simulink model "sampleModel185"  (R2021b)
settings: Solver=VariableStepAuto  StartTime=0.0  StopTime=10.0  RelTol=1e-3
undefined symbols (not defined in the file or in its folder): DiscIntNeverNeededParam, Newton, Raphson
libraries: simulink x18, slpidlib x1
settings Model: Creator=user  LastModifiedBy=user

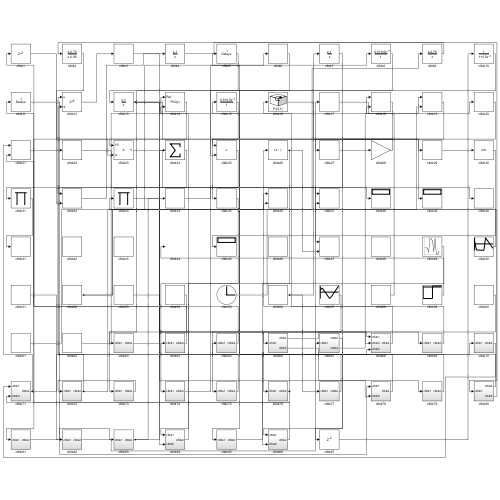
[thumbnail: Simulink's stored preview of the top-level diagram]
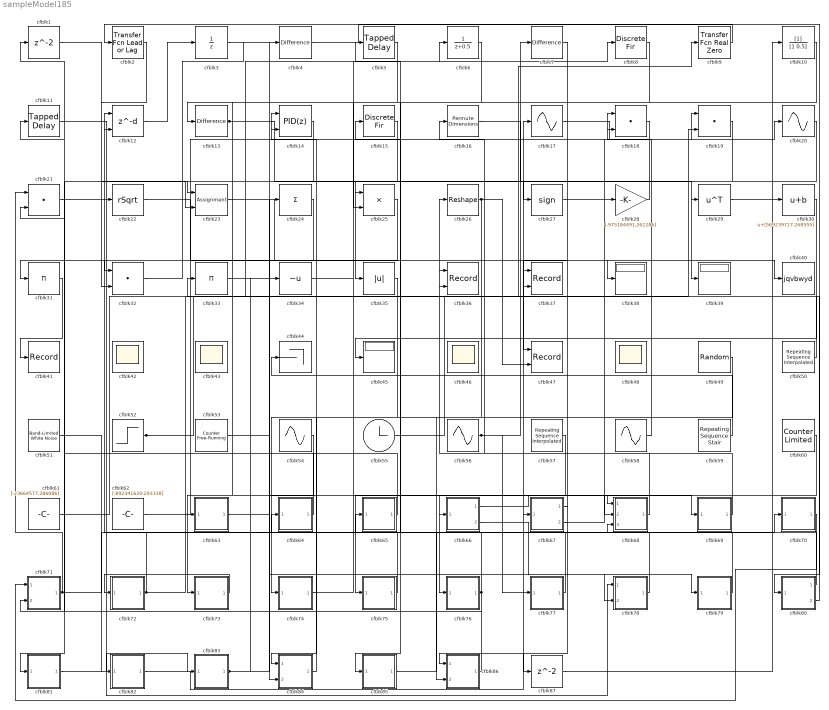
== system sampleModel185 ==
  cfblk1 : Delay  SampleTime=1
  cfblk10 : DiscreteFilter  SampleTime=1
  cfblk11 : simulink/Discrete/Tapped Delay  vinit=0.0  samptime=-1  NumDelays=1  DelayOrder=Oldest  includeCurrent=off
  cfblk12 : Delay  DelayLengthSource=Input port  SampleTime=1
      settings: InputPortMap=u0,p1
  cfblk13 : simulink/Discrete/Difference  ICPrevInput=0.0  OutMin=[]  OutMax=[]  OutDataTypeStr=Inherit: Inherit via back propagation  OutDataType=fixdt(1, 16)  OutScaling=2^-10  DoSatur=off
  cfblk14 : slpidlib/PID Controller (2DOF)  Controller=PID  Form=Parallel  TimeDomain=Discrete-time  UseExternalTs=off  SampleTime=1  IntegratorMethod=Forward Euler  FilterMethod=Forward Euler  ControllerParametersSource=internal  P=1  I=1  D=0  UseFilter=on  N=100  b=1  c=1  TunerSelectOption=Transfer Function Based (PID Tuner App)  InitialConditionSource=internal  InitialConditionForIntegrator=0  InitialConditionForFilter=0  DifferentiatorICPrevScaledInput=0  ExternalReset=none  TrackingMode=off  Kt=1  LimitOutput=off  SatLimitsSource=internal  UpperSaturationLimit=inf  LowerSaturationLimit=-inf  LinearizeAsGain=off  AntiWindupMode=none  Kb=1  POutMin=[]  POutMax=[]  IOutMin=[]  IOutMax=[]  DOutMin=[]  DOutMax=[]  NOutMin=[]  NOutMax=[]  bOutMin=[]  bOutMax=[]  cOutMin=[]  cOutMax=[]  SumOutMin=[]  SumOutMax=[]  SaturationOutMin=[]  SaturationOutMax=[]  PParamMin=[]  PParamMax=[]  IParamMin=[]  IParamMax=[]  DParamMin=[]  DParamMax=[]  NParamMin=[]  NParamMax=[]  bParamMin=[]  bParamMax=[]  cParamMin=[]  cParamMax=[]  KbParamMin=[]  KbParamMax=[]  KtParamMin=[]  KtParamMax=[]  KbOutMin=[]  KbOutMax=[]  KtOutMin=[]  KtOutMax=[]  IntegratorOutMin=[]  IntegratorOutMax=[]  FilterOutMin=[]  FilterOutMax=[]  SumI1OutMin=[]  SumI1OutMax=[]  SumI2OutMin=[]  SumI2OutMax=[]  SumI3OutMin=[]  SumI3OutMax=[]  SumI4OutMin=[]  SumI4OutMax=[]  SumDOutMin=[]  SumDOutMax=[]  Sum1OutMin=[]  Sum1OutMax=[]  Sum2OutMin=[]  Sum2OutMax=[]  Sum3OutMin=[]  Sum3OutMax=[]  DifferentiatorOutMin=[]  DifferentiatorOutMax=[]  FilterDiffOutCoefMin=[]  FilterDiffOutCoefMax=[]  ReciprocalOutMin=[]  ReciprocalOutMax=[]  SumDenOutMin=[]  SumDenOutMax=[]  SumNumOutMin=[]  SumNumOutMax=[]  DivideOutMin=[]  DivideOutMax=[]  UdiffTsProdOutMin=[]  UdiffTsProdOutMax=[]  NTsProdOutMin=[]  NTsProdOutMax=[]  UintegralTsProdOutMin=[]  UintegralTsProdOutMax=[]  UngainTsProdOutMin=[]  UngainTsProdOutMax=[]  IntegratorContinuousStateAttributes=''  IntegratorStateMustResolveToSignalObject=off  IntegratorRTWStateStorageClass=Auto  FilterContinuousStateAttributes=''  FilterStateMustResolveToSignalObject=off  FilterRTWStateStorageClass=Auto  ParallelPVariant=InternalParameters  IdealPVariant=Disabled  IVariant=InternalParameters  DVariant=InternalParameters  bVariant=InternalParameters  cVariant=InternalParameters  IntegratorVariant=Discrete  SatVariant=Disabled  AWVariant=Passthrough  PCopyVariant=Disabled  TRVariant=Disabled  FdbkBlocksVariant=Forward  IdealPFdbkVariant=Disabled  SatFdbkVariant=Disabled  DerivativeFilterVariant=ForwardEulerFilter  NVariant=InternalParameters  NCopyVariant=Disabled  FilterICVariant=InternalICsFilter  IntegratorICVariant=InternalICs  ExternalResetVariant=Disabled  TRSumVariant=Passthrough  SumFdbkVariant=Disabled  SumVariant=Sum_PID  TsampFilterVariant=InternalTs  TsampNgainVariant=Passthrough  TsampIntegralVariant=Passthrough  ExternalSaturationOutDataTypeStr=Inherit: Same as second input
      settings: SourceProductBaseCode=SL
  cfblk15 : DiscreteFir  SampleTime=1
  cfblk16 : PermuteDimensions
  cfblk17 : Sin  TimeSource=Use external signal  SampleTime=0
  cfblk{18..19,21,32} (4 alike) : DotProduct  InputSameDT=on  OutDataTypeStr=Inherit: Inherit via internal rule
  cfblk2 : simulink/Discrete/Transfer Fcn Lead or Lag  PoleZ=0.95  ZeroZ=0.75  ICPrevOutput=0.0  ICPrevInput=0.0  DoSatur=off
      settings: SourceProductBaseCode=SL
  cfblk20 : Sin  TimeSource=Use external signal  SampleTime=0
  cfblk22 : Sqrt  Operator=rSqrt  AlgorithmType=Newton-Raphson  SaturateOnIntegerOverflow=on
  cfblk23 : Assignment  DiagnosticForDimensions=Warning  IndexOptions=Index vector (dialog)  Indices=1  OutputSizes=1
  cfblk24 : Sum  Inputs=+
  cfblk25 : Product
  cfblk26 : Reshape
  cfblk27 : Signum
  cfblk28 : Gain  Gain=[-975184491.261286]
  cfblk29 : Math  Operator=transpose  SaturateOnIntegerOverflow=on
  cfblk3 : UnitDelay  HasFrameUpgradeWarning=on
  cfblk30 : Bias  Bias=[569239717.268555]
  cfblk31 : Product  Inputs=*
  cfblk33 : Product  Inputs=*
  cfblk34 : UnaryMinus
  cfblk35 : Abs
  cfblk36 : Record  FileSettingsInternal="{\"entries\":[{\"content\":{\"excelSettings\":{\"content\":{},\"type\":\"Streamout.ExcelSettings\"}},\"type\":\"Streamout.FileSettingStorage\",\"uuid\":\"ca3dc4c8-2701-4d7d-a74f-2876e6223ae4\"}],\"packageUris\":[\"http://schema.mathworks.com/mf0/streamout_blocks/R2020a\"],\"version\":\"1.0\"}"  Layout=[1 1]  SignalsInternal="{\"entries\":[{\"content\":{\"signals\":[{\"content\":{\"blockPath\":[\"sampleModel185/cfblk36\"],\"channel\":[],\"dimensions\":[1],\"domain\":\"sampleModel185/cfblk36\",\"lineColor\":\"#a2142f\",\"plots\":[1],\"port\":1,\"sid\":[\"\"],\"signalID\":6898,\"signalName\":\"cfblk83\"},\"type\":\"RecordBlkView.Signal\",\"uuid\":\"58bfe43f-3551-43b7-ad72-a19eb20e3563\"},{\"content\":{\"blockPath\":[\"sampleModel185/cfblk36\"],\"channel\":[],\"dimensions\":[1],\"domain\":\"sampleModel185/cfblk36\",\"lineColor\":\"#139fff\",\"plots\":[1],\"port\":2,\"sid\":[\"\"],\"signalID\":6902,\"signalName\":\"cfblk72\"},\"type\":\"RecordBlkView.Signal\",\"uuid\":\"e367b23f-37ad-4773-b756-b56c609fc008\"}]},\"type\":\"RecordBlkView.InputSignals\",\"uuid\":\"b769fd5a-4ead-4659-9e0d-ec7d5ec301cf\"}],\"packageUris\":[\"http://schema.mathworks.com/mf0/streamout_blocks/R2020a\"],\"version\":\"1.0\"}"  VisualizationBindings="{\"xyplotplugin\":{\"info\":[{\"series\":[{\"bindingParametersList\":[{\"parameter\":\"X-Axis\",\"signalID\":6898,\"signalName\":\"cfblk83\"},{\"parameter\":\"Y-Axis\",\"signalID\":6902,\"signalName\":\"cfblk72\"}],\"seriesID\":54905}],\"subplotID\":1}]}}"  CompatibilityTag=XY
  cfblk37 : Record  FileSettingsInternal="{\"entries\":[{\"content\":{\"excelSettings\":{\"content\":{},\"type\":\"Streamout.ExcelSettings\"}},\"type\":\"Streamout.FileSettingStorage\",\"uuid\":\"82f9f1e3-03ac-43a3-94a3-1711c234262c\"}],\"packageUris\":[\"http://schema.mathworks.com/mf0/streamout_blocks/R2020a\"],\"version\":\"1.0\"}"  Layout=[1 1]  SignalsInternal="{\"entries\":[{\"content\":{\"signals\":[{\"content\":{\"blockPath\":[\"sampleModel185/cfblk37\"],\"channel\":[],\"dimensions\":[1],\"domain\":\"sampleModel185/cfblk37\",\"lineColor\":\"#a2142f\",\"plots\":[1],\"port\":1,\"sid\":[\"\"],\"signalID\":6906,\"signalName\":\"cfblk7\"},\"type\":\"RecordBlkView.Signal\",\"uuid\":\"5167ba9e-1071-42f9-84ca-5e71217b0861\"},{\"content\":{\"blockPath\":[\"sampleModel185/cfblk37\"],\"channel\":[],\"dimensions\":[1,1],\"domain\":\"sampleModel185/cfblk37\",\"lineColor\":\"#139fff\",\"plots\":[1],\"port\":2,\"sid\":[\"\"],\"signalID\":6910,\"signalName\":\"cfblk80:2\"},\"type\":\"RecordBlkView.Signal\",\"uuid\":\"c3a57a63-0921-4f5f-8c56-e80736f511fc\"}]},\"type\":\"RecordBlkView.InputSignals\",\"uuid\":\"116cf8fd-94b0-4b46-9554-bd59143511f7\"}],\"packageUris\":[\"http://schema.mathworks.com/mf0/streamout_blocks/R2020a\"],\"version\":\"1.0\"}"  VisualizationBindings="{\"xyplotplugin\":{\"info\":[{\"series\":[{\"bindingParametersList\":[{\"parameter\":\"X-Axis\",\"signalID\":6906,\"signalName\":\"cfblk7\"},{\"parameter\":\"Y-Axis\",\"signalID\":6910,\"signalName\":\"cfblk80:2\"}],\"seriesID\":58278}],\"subplotID\":1}]}}"  CompatibilityTag=XY
  cfblk38 : Display
  cfblk39 : Display
  cfblk4 : simulink/Discrete/Difference  ICPrevInput=0.0  OutMin=[]  OutMax=[]  OutDataTypeStr=Inherit: Inherit via back propagation  OutDataType=fixdt(1, 16)  OutScaling=2^-10  DoSatur=off
  cfblk40 : ToWorkspace  VariableName=jqvbwyd  SaveFormat=Timeseries  SampleTime=-1
  cfblk41 : Record  FileSettingsInternal="{\"entries\":[{\"content\":{\"excelSettings\":{\"content\":{},\"type\":\"Streamout.ExcelSettings\"}},\"type\":\"Streamout.FileSettingStorage\",\"uuid\":\"d4802ba6-05bd-4ddf-8b8e-f99e9f8eb8d9\"}],\"packageUris\":[\"http://schema.mathworks.com/mf0/streamout_blocks/R2020a\"],\"version\":\"1.0\"}"  SignalsInternal="{\"entries\":[{\"content\":{\"signals\":[{\"content\":{\"blockPath\":[\"sampleModel185/cfblk41\"],\"channel\":[],\"dimensions\":[1],\"domain\":\"sampleModel185/cfblk41\",\"lineColor\":\"#77ac30\",\"plots\":[1],\"port\":1,\"sid\":[\"\"],\"signalID\":6922,\"signalName\":\"cfblk31\"},\"type\":\"RecordBlkView.Signal\",\"uuid\":\"55ffb5aa-6727-4748-88e1-27207a70595c\"}]},\"type\":\"RecordBlkView.InputSignals\",\"uuid\":\"a3da5140-dce7-4d31-869c-5c8311695e55\"}],\"packageUris\":[\"http://schema.mathworks.com/mf0/streamout_blocks/R2020a\"],\"version\":\"1.0\"}"  VisualizationBindings="{\"sparklinesplugin\":{\"info\":[{\"bindingParametersList\":[],\"subplotID\":1}]}}"
  cfblk{42..43,46,48} (4 alike) : Scope
      settings: Floating=on
  cfblk44 : Terminator
  cfblk45 : Display
  cfblk47 : Record  FileSettingsInternal="{\"entries\":[{\"content\":{\"excelSettings\":{\"content\":{},\"type\":\"Streamout.ExcelSettings\"}},\"type\":\"Streamout.FileSettingStorage\",\"uuid\":\"3a4413fc-1f12-4c68-bc16-d515da000100\"}],\"packageUris\":[\"http://schema.mathworks.com/mf0/streamout_blocks/R2020a\"],\"version\":\"1.0\"}"  Layout=[1 1]  SignalsInternal="{\"entries\":[{\"content\":{\"signals\":[{\"content\":{\"blockPath\":[\"sampleModel185/cfblk47\"],\"channel\":[],\"dimensions\":[1],\"domain\":\"sampleModel185/cfblk47\",\"lineColor\":\"#a2142f\",\"plots\":[1],\"port\":1,\"sid\":[\"\"],\"signalID\":6914,\"signalName\":\"cfblk22\"},\"type\":\"RecordBlkView.Signal\",\"uuid\":\"415c6105-a7e5-4e59-83e1-d8c7c00c7edb\"},{\"content\":{\"blockPath\":[\"sampleModel185/cfblk47\"],\"channel\":[],\"dimensions\":[1],\"domain\":\"sampleModel185/cfblk47\",\"lineColor\":\"#139fff\",\"plots\":[1],\"port\":2,\"sid\":[\"\"],\"signalID\":6918,\"signalName\":\"cfblk26\"},\"type\":\"RecordBlkView.Signal\",\"uuid\":\"650bcf49-f9e2-4cd9-ba28-49d1076f9c6e\"}]},\"type\":\"RecordBlkView.InputSignals\",\"uuid\":\"a6998b43-a6f9-4b13-bd8b-626c6ffd083e\"}],\"packageUris\":[\"http://schema.mathworks.com/mf0/streamout_blocks/R2020a\"],\"version\":\"1.0\"}"  VisualizationBindings="{\"xyplotplugin\":{\"info\":[{\"series\":[{\"bindingParametersList\":[{\"parameter\":\"X-Axis\",\"signalID\":6914,\"signalName\":\"cfblk22\"},{\"parameter\":\"Y-Axis\",\"signalID\":6918,\"signalName\":\"cfblk26\"}],\"seriesID\":35509}],\"subplotID\":1}]}}"  CompatibilityTag=XY
  cfblk49 : RandomNumber  Mean=[22057.459232]  Variance=[14627.121236]  Seed=[908376181.000000]  SampleTime=0.1
  cfblk5 : simulink/Discrete/Tapped Delay  vinit=0.0  samptime=-1  NumDelays=1  DelayOrder=Oldest  includeCurrent=off
  cfblk50 : simulink/Sources/Repeating Sequence Interpolated  OutValues=[327193278.074177, -826175416.820414, -852348471.400204, 802852631.601716, -603146606.256838]  TimeValues=[0 0.1 0.5 0.6 1].'  LookUpMeth=Interpolation-Use End Values  tsamp=0.01  OutMin=[]  OutMax=[]  OutDataTypeStr=double  OutputDataTypeScalingMode=double  OutDataType=fixdt(0,8)  OutScaling=2^-10
  cfblk51 : simulink/Sources/Band-Limited White Noise  Cov=[6799802650.188495]  Ts=0.1  seed=[5355830120.000000]
  cfblk52 : Step  Time=[21.000000]  Before=[-839865693.190419]  After=[-28942891.132493]  SampleTime=0
  cfblk53 : simulink/Sources/Counter Free-Running  NumBits=[23.000000]  tsamp=-1
  cfblk54 : Sin  Amplitude=[-493649667.444895]  Bias=[372403373.682373]  SampleTime=0
  cfblk55 : Clock
  cfblk56 : Sin  Amplitude=[-692553084.611350]  Bias=[847742899.509054]  SampleTime=0
  cfblk57 : simulink/Sources/Repeating Sequence Interpolated  OutValues=[241508202.351314, 580090238.893388, -869366063.798662, -680391875.863791, 843444654.744957]  TimeValues=[0 0.1 0.5 0.6 1].'  LookUpMeth=Use Input Above  tsamp=0.01  OutMin=[]  OutMax=[]  OutDataTypeStr=double  OutputDataTypeScalingMode=double  OutDataType=fixdt(0,8)  OutScaling=2^-10
  cfblk58 : Sin  Amplitude=[-442584007.207837]  Bias=[832753916.372387]  SampleTime=0
  cfblk59 : simulink/Sources/Repeating Sequence Stair  OutValues=[-937317867.234295, 88035866.976802]  tsamp=-1  OutMin=[]  OutMax=[]  OutDataTypeStr=double  OutputDataTypeScalingMode=double  OutDataType=fixdt(0,8)  ConRadixGroup=Best Precision: Vector-wise  OutScaling=2^-12
  cfblk6 : DiscreteTransferFcn  SampleTime=1
  cfblk60 : simulink/Sources/Counter Limited  uplimit=[750.000000]  tsamp=-1
  cfblk61 : Constant  Value=[-23664577.286086]  SampleTime=1
  cfblk62 : Constant  Value=[-892341620.293338]  SampleTime=1
  cfblk63 : Subsystem
  cfblk64 : Subsystem
  cfblk65 : Subsystem
  cfblk66 : Subsystem
  cfblk67 : Subsystem
  cfblk68 : Subsystem
  cfblk69 : Subsystem
  cfblk7 : simulink/Discrete/Difference  ICPrevInput=0.0  OutMin=[]  OutMax=[]  OutDataTypeStr=Inherit: Inherit via back propagation  OutDataType=fixdt(1, 16)  OutScaling=2^-10  DoSatur=off
  cfblk70 : Subsystem
  cfblk71 : Subsystem
  cfblk72 : Subsystem
  cfblk73 : Subsystem
  cfblk74 : Subsystem
  cfblk75 : Subsystem
  cfblk76 : Subsystem
  cfblk77 : Subsystem
  cfblk78 : Subsystem
  cfblk79 : Subsystem
  cfblk8 : DiscreteFir  SampleTime=1
  cfblk80 : Subsystem
  cfblk81 : Subsystem
  cfblk82 : Subsystem
  cfblk83 : Subsystem
  cfblk84 : Subsystem
  cfblk85 : Subsystem
  cfblk86 : Subsystem
  cfblk87 : Delay  SampleTime=1
  cfblk9 : simulink/Discrete/Transfer Fcn Real Zero  ZeroZ=0.75  ICPrevInput=0.0  DoSatur=off
      settings: SourceProductBaseCode=SL
  wires:
  cfblk31/1 -> cfblk41/1
  cfblk83/1(cfblk2) -> cfblk34/1, cfblk36/1
  cfblk52/1 -> cfblk8/1, cfblk19/2
  cfblk82/1(cfblk2) -> cfblk17/1
  cfblk62/1 -> cfblk14/1
  cfblk55/1 -> cfblk9/1
  cfblk57/1 -> cfblk75/1(cfblk1)
  cfblk11/1 -> cfblk78/1(cfblk1)
  cfblk66/1(cfblk2) -> cfblk69/1(cfblk1)
  cfblk23/1 -> cfblk38/1
  cfblk54/1 -> cfblk73/1(cfblk1)
  cfblk50/1 -> cfblk33/1
  cfblk15/1 -> cfblk35/1
  cfblk20/1 -> cfblk27/1
  cfblk26/1 -> cfblk74/1(cfblk1), cfblk47/2
  cfblk21/1 -> cfblk12/1
  cfblk56/1 -> cfblk7/1, cfblk77/1(cfblk1)
  cfblk61/1 -> cfblk24/1
  cfblk84/1(cfblk2) -> cfblk64/1(cfblk1)
  cfblk73/1(cfblk2) -> cfblk72/1(cfblk1)
  cfblk32/1 -> cfblk4/1
  cfblk69/1(cfblk2) -> cfblk26/1
  cfblk35/1 -> cfblk84/1(cfblk1)
  cfblk24/1 -> cfblk81/1(cfblk1)
  cfblk60/1 -> cfblk76/1(cfblk1)
  cfblk19/1 -> cfblk23/1
  cfblk67/1(cfblk2) -> cfblk86/1(cfblk1)
  cfblk65/1(cfblk2) -> cfblk1/1
  cfblk77/1(cfblk2) -> cfblk12/2
  cfblk5/1 -> cfblk63/1(cfblk1)
  cfblk71/1(cfblk2) -> cfblk21/1, cfblk68/3(cfblk5)
  cfblk72/1(cfblk2) -> cfblk22/1, cfblk36/2
  cfblk81/1(cfblk2) -> cfblk83/1(cfblk1)
  cfblk13/1 -> cfblk39/1, cfblk78/2(cfblk5), cfblk18/2
  cfblk66/2(cfblk5) -> cfblk79/1(cfblk1)
  cfblk68/1(cfblk2) -> cfblk16/1
  cfblk16/1 -> cfblk29/1
  cfblk74/1(cfblk2) -> cfblk6/1
  cfblk4/1 -> cfblk80/1(cfblk1)
  cfblk64/1(cfblk2) -> cfblk21/2
  cfblk28/1 -> cfblk25/1
  cfblk34/1 -> cfblk40/1
  cfblk85/1(cfblk2) -> cfblk70/1(cfblk1)
  cfblk78/1(cfblk2) -> cfblk5/1
  cfblk63/1(cfblk2) -> cfblk68/1(cfblk1)
  cfblk3/1 -> cfblk66/1(cfblk1)
  cfblk12/1 -> cfblk3/1
  cfblk79/1(cfblk2) -> cfblk44/1
  cfblk10/1 -> cfblk13/1
  cfblk6/1 -> cfblk25/2
  cfblk30/1 -> cfblk45/1
  cfblk70/1(cfblk2) -> cfblk71/1(cfblk1)
  cfblk86/1(cfblk2) -> cfblk11/1
  cfblk59/1 -> cfblk14/2
  cfblk27/1 -> cfblk28/1
  cfblk14/1 -> cfblk31/1
  cfblk51/1 -> cfblk82/1(cfblk1)
  cfblk29/1 -> cfblk30/1
  cfblk53/1 -> cfblk84/2(cfblk5)
  cfblk49/1 -> cfblk86/2(cfblk4)
  cfblk9/1 -> cfblk2/1
  cfblk58/1 -> cfblk18/1
  cfblk80/1(cfblk2) -> cfblk67/1(cfblk1)
  cfblk17/1 -> cfblk20/1
  cfblk25/1 -> cfblk32/1
  cfblk76/1(cfblk2) -> cfblk71/2(cfblk3), cfblk15/1
  cfblk22/1 -> cfblk47/1
  cfblk8/1 -> cfblk85/1(cfblk1)
  cfblk2/1 -> cfblk32/2
  cfblk75/1(cfblk2) -> cfblk65/1(cfblk1)
  cfblk1/1 -> cfblk23/2
  cfblk7/1 -> cfblk37/1
  cfblk80/2(cfblk5) -> cfblk37/2
  cfblk33/1 -> cfblk68/2(cfblk4)
  cfblk67/2(cfblk4) -> cfblk19/1
  cfblk18/1 -> cfblk87/1
  cfblk87/1 -> cfblk10/1

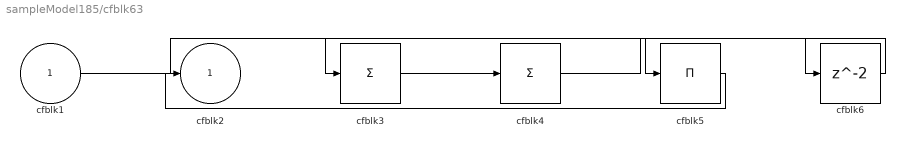
== system sampleModel185/cfblk63 ==
  cfblk1 : Inport
  cfblk3 : Sum  Inputs=+
  cfblk4 : Sum  Inputs=+
  cfblk5 : Product  Inputs=*
  cfblk6 : Delay  SampleTime=1
  cfblk2 : Outport
  wires:
  cfblk1/1 -> cfblk5/1
  cfblk5/1 -> cfblk2/1
  cfblk3/1 -> cfblk4/1
  cfblk4/1 -> cfblk6/1
  cfblk6/1 -> cfblk3/1

== system sampleModel185/cfblk64 ==
  cfblk1 : Inport
  cfblk3 : Constant  Value=[796212373.254412]  SampleTime=1
  cfblk2 : Outport
  wires:
  cfblk3/1 -> cfblk2/1

== system sampleModel185/cfblk65 ==
  cfblk1 : Inport
  cfblk3 : Trigonometry
  cfblk2 : Outport
  wires:
  cfblk1/1 -> cfblk3/1
  cfblk3/1 -> cfblk2/1

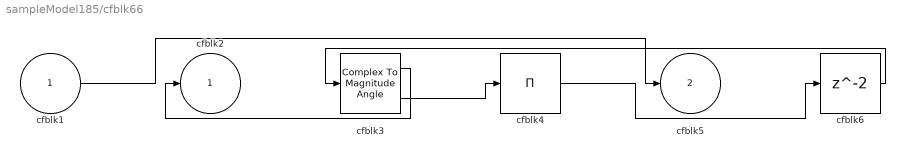
== system sampleModel185/cfblk66 ==
  cfblk1 : Inport
  cfblk3 : ComplexToMagnitudeAngle
  cfblk4 : Product  Inputs=*
  cfblk6 : Delay  SampleTime=1
  cfblk2 : Outport
  cfblk5 : Outport  Port=2
  wires:
  cfblk3/1 -> cfblk2/1
  cfblk3/2 -> cfblk4/1
  cfblk1/1 -> cfblk5/1
  cfblk4/1 -> cfblk6/1
  cfblk6/1 -> cfblk3/1

== system sampleModel185/cfblk67 ==
  cfblk1 : Inport
  cfblk3 : Constant  Value=[-880603735.218664]  SampleTime=1
  cfblk2 : Outport
  cfblk4 : Outport  Port=2
  wires:
  cfblk1/1 -> cfblk2/1
  cfblk3/1 -> cfblk4/1

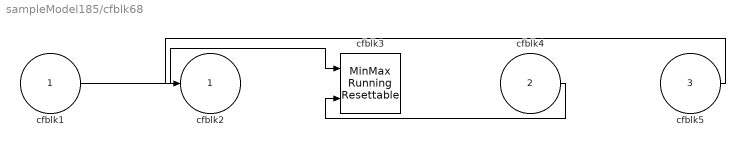
== system sampleModel185/cfblk68 ==
  cfblk1 : Inport
  cfblk4 : Inport  Port=2
  cfblk5 : Inport  Port=3
  cfblk3 : simulink/Math Operations/MinMax Running Resettable  Function=min  vinit=0.0
  cfblk2 : Outport
  wires:
  cfblk1/1 -> cfblk3/1
  cfblk4/1 -> cfblk3/2
  cfblk5/1 -> cfblk2/1

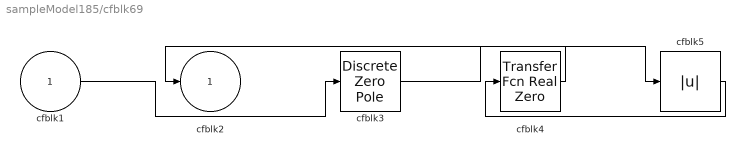
== system sampleModel185/cfblk69 ==
  cfblk1 : Inport
  cfblk3 : DiscreteZeroPole  Poles=[0 0.5]  Gain=1
  cfblk4 : simulink/Discrete/Transfer Fcn Real Zero  ZeroZ=0.75  ICPrevInput=0.0  DoSatur=off
      settings: SourceProductBaseCode=SL
  cfblk5 : Abs
  cfblk2 : Outport
  wires:
  cfblk4/1 -> cfblk2/1
  cfblk5/1 -> cfblk4/1
  cfblk3/1 -> cfblk5/1
  cfblk1/1 -> cfblk3/1

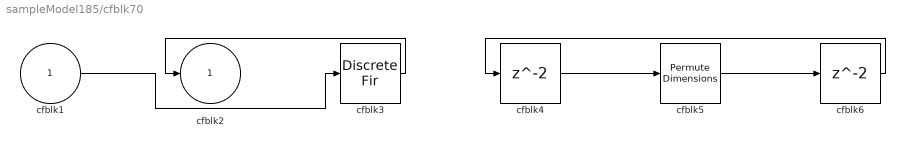
== system sampleModel185/cfblk70 ==
  cfblk1 : Inport
  cfblk3 : DiscreteFir  SampleTime=1
  cfblk4 : Delay  SampleTime=1
  cfblk5 : PermuteDimensions
  cfblk6 : Delay  SampleTime=1
  cfblk2 : Outport
  wires:
  cfblk3/1 -> cfblk2/1
  cfblk4/1 -> cfblk5/1
  cfblk1/1 -> cfblk3/1
  cfblk5/1 -> cfblk6/1
  cfblk6/1 -> cfblk4/1

== system sampleModel185/cfblk71 ==
  cfblk1 : Inport
  cfblk3 : Inport  Port=2
  cfblk2 : Outport
  wires:
  cfblk1/1 -> cfblk2/1

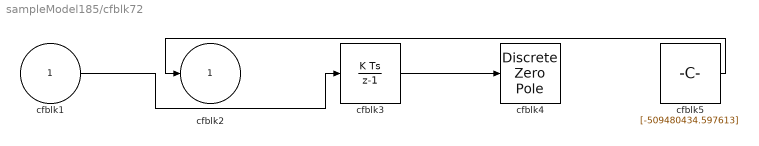
== system sampleModel185/cfblk72 ==
  cfblk1 : Inport
  cfblk3 : DiscreteIntegrator  ICPrevOutput=DiscIntNeverNeededParam  ICPrevScaledInput=DiscIntNeverNeededParam
  cfblk4 : DiscreteZeroPole  Poles=[0 0.5]  Gain=1
  cfblk5 : Constant  Value=[-509480434.597613]  SampleTime=1
  cfblk2 : Outport
  wires:
  cfblk5/1 -> cfblk2/1
  cfblk1/1 -> cfblk3/1
  cfblk3/1 -> cfblk4/1

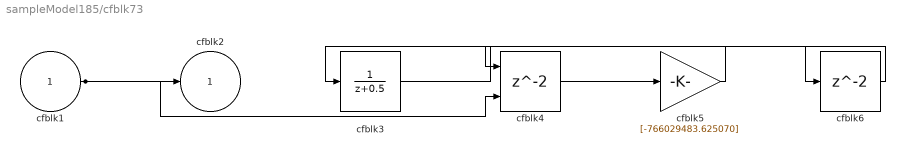
== system sampleModel185/cfblk73 ==
  cfblk1 : Inport
  cfblk3 : DiscreteTransferFcn  SampleTime=1
  cfblk4 : Delay  ShowEnablePort=on  SampleTime=1
      settings: InputPortMap=u0,e6
  cfblk5 : Gain  Gain=[-766029483.625070]
  cfblk6 : Delay  SampleTime=1
  cfblk2 : Outport
  wires:
  cfblk5/1 -> cfblk3/1
  cfblk1/1 -> cfblk2/1, cfblk4/2
  cfblk4/1 -> cfblk5/1
  cfblk3/1 -> cfblk6/1
  cfblk6/1 -> cfblk4/1

== system sampleModel185/cfblk74 ==
  cfblk1 : Inport
  cfblk3 : Sum  Inputs=|++
  cfblk2 : Outport
  wires:
  cfblk1/1 -> cfblk2/1, cfblk3/1, cfblk3/2

== system sampleModel185/cfblk75 ==
  cfblk1 : Inport
  cfblk3 : simulink/Discrete/Transfer Fcn Lead or Lag  PoleZ=0.95  ZeroZ=0.75  ICPrevOutput=0.0  ICPrevInput=0.0  DoSatur=off
      settings: SourceProductBaseCode=SL
  cfblk2 : Outport
  wires:
  cfblk3/1 -> cfblk2/1
  cfblk1/1 -> cfblk3/1

== system sampleModel185/cfblk76 ==
  cfblk1 : Inport
  cfblk3 : UnitDelay  HasFrameUpgradeWarning=on
  cfblk2 : Outport
  wires:
  cfblk1/1 -> cfblk3/1
  cfblk3/1 -> cfblk2/1

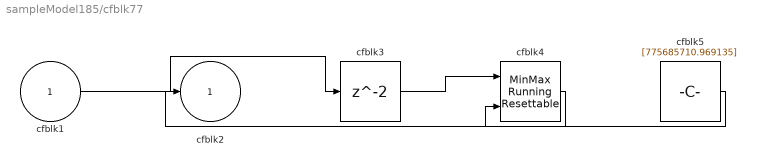
== system sampleModel185/cfblk77 ==
  cfblk1 : Inport
  cfblk3 : Delay  SampleTime=1
  cfblk4 : simulink/Math Operations/MinMax Running Resettable  Function=min  vinit=0.0
  cfblk5 : Constant  Value=[775685710.969135]  SampleTime=1
  cfblk2 : Outport
  wires:
  cfblk3/1 -> cfblk4/1
  cfblk1/1 -> cfblk3/1
  cfblk4/1 -> cfblk2/1
  cfblk5/1 -> cfblk4/2

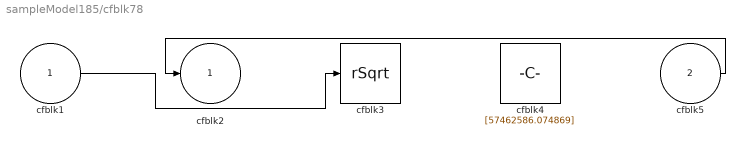
== system sampleModel185/cfblk78 ==
  cfblk1 : Inport
  cfblk5 : Inport  Port=2
  cfblk3 : Sqrt  Operator=rSqrt  AlgorithmType=Newton-Raphson  SaturateOnIntegerOverflow=on
  cfblk4 : Constant  Value=[57462586.074869]  SampleTime=1
  cfblk2 : Outport
  wires:
  cfblk5/1 -> cfblk2/1
  cfblk1/1 -> cfblk3/1

== system sampleModel185/cfblk79 ==
  cfblk1 : Inport
  cfblk3 : DiscreteStateSpace
  cfblk2 : Outport
  wires:
  cfblk1/1 -> cfblk2/1, cfblk3/1

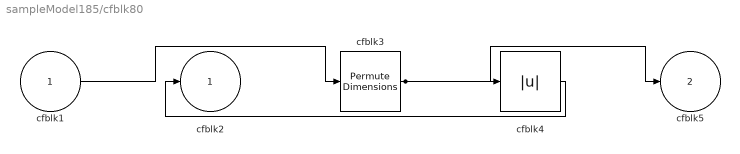
== system sampleModel185/cfblk80 ==
  cfblk1 : Inport
  cfblk3 : PermuteDimensions
  cfblk4 : Abs
  cfblk2 : Outport
  cfblk5 : Outport  Port=2
  wires:
  cfblk3/1 -> cfblk5/1, cfblk4/1
  cfblk4/1 -> cfblk2/1
  cfblk1/1 -> cfblk3/1

== system sampleModel185/cfblk81 ==
  cfblk1 : Inport
  cfblk3 : Signum
  cfblk4 : MinMax  Function=max  Inputs=3
  cfblk5 : Constant  Value=[-7546107.891919]  SampleTime=1
  cfblk2 : Outport
  wires:
  cfblk3/1 -> cfblk4/1, cfblk4/3
  cfblk4/1 -> cfblk2/1
  cfblk1/1 -> cfblk4/2
  cfblk5/1 -> cfblk3/1

== system sampleModel185/cfblk82 ==
  cfblk1 : Inport
  cfblk3 : DiscreteFilter  SampleTime=1
  cfblk4 : Sum  Inputs=--
  cfblk5 : Delay  SampleTime=1
  cfblk2 : Outport
  wires:
  cfblk4/1 -> cfblk3/1
  cfblk1/1 -> cfblk4/1, cfblk2/1
  cfblk3/1 -> cfblk5/1
  cfblk5/1 -> cfblk4/2

== system sampleModel185/cfblk83 ==
  cfblk1 : Inport
  cfblk3 : simulink/Math Operations/Slider Gain  gain=1  low=0  high=2
  cfblk2 : Outport
  wires:
  cfblk1/1 -> cfblk2/1, cfblk3/1

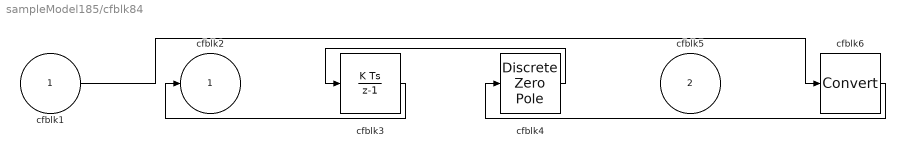
== system sampleModel185/cfblk84 ==
  cfblk1 : Inport
  cfblk5 : Inport  Port=2
  cfblk3 : DiscreteIntegrator  ICPrevOutput=DiscIntNeverNeededParam  ICPrevScaledInput=DiscIntNeverNeededParam
  cfblk4 : DiscreteZeroPole  Poles=[0 0.5]  Gain=1
  cfblk6 : DataTypeConversion
  cfblk2 : Outport
  wires:
  cfblk4/1 -> cfblk3/1
  cfblk3/1 -> cfblk2/1
  cfblk1/1 -> cfblk6/1
  cfblk6/1 -> cfblk4/1

== system sampleModel185/cfblk85 ==
  cfblk1 : Inport
  cfblk3 : DiscreteFir  SampleTime=1
  cfblk4 : Abs
  cfblk2 : Outport
  wires:
  cfblk1/1 -> cfblk4/1
  cfblk4/1 -> cfblk2/1, cfblk3/1

== system sampleModel185/cfblk86 ==
  cfblk1 : Inport
  cfblk4 : Inport  Port=2
  cfblk3 : Product  Inputs=**
  cfblk2 : Outport
  wires:
  cfblk1/1 -> cfblk3/1, cfblk3/2
  cfblk4/1 -> cfblk2/1
